simulink library "flight_dynamics_models"  (R2018b)
settings: Solver=VariableStepAuto  StartTime=0.0  StopTime=10.0  RelTol=1e-3
undefined symbols (not defined in the file or in its folder): aircraft, ic
libraries: vlm_wing_lib x12, flight_parameters_lib x4, axes_transformation_lib x4, fuselage_lib x4, wing_downwash_lib x4, se2a_actuators_lib x4, $bdroot x2, flexibleBody_lib x2, rigidBody_lib x2
(part 1 of 2)
settings Model: Creator=Ybeyer  LastModifiedBy=yannic
settings SFSimCC: SimUseLocalCustomCode=off
settings RTWCC: RTWUseLocalCustomCode=off
settings CodeAppCC: StateflowObjectComments=on

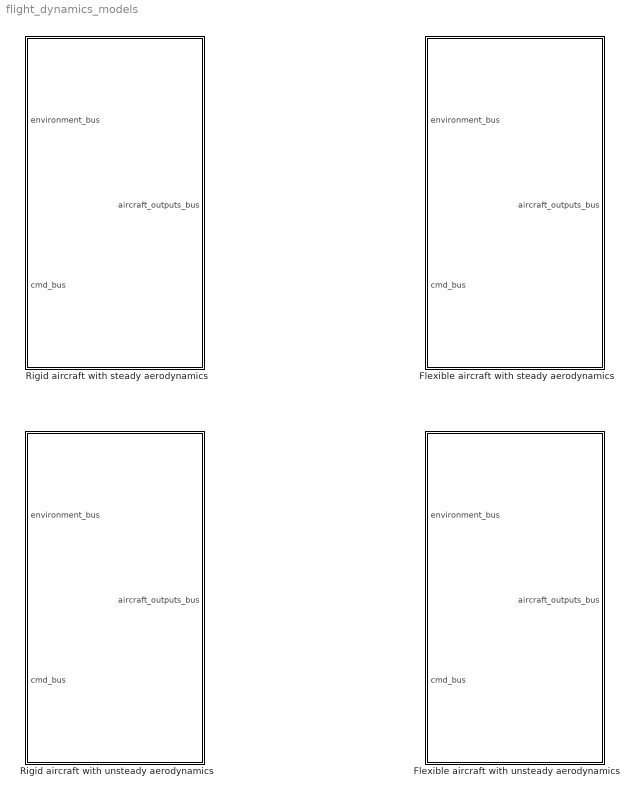
== system flight_dynamics_models ==
  Flexible aircraft with steady aerodynamics : Subsystem  mask{aircraft=aircraft, ic=ic}
      mask prompts: aircraft "Aircraft parameters struct, see aircraftSe2aCreate"; ic "Initial conditions struct"
      mask init:
      | aircraft_state = aircraftSe2aGetState(aircraft);
      | struct2bus(aircraft_state);
      mask DialogControl DescGroupVar Prompt: Rigid aircraft with steady aerodynamics
      mask DialogControl DescTextVar Prompt: Rigid body aerodynamics, steady aerodynamics based on nonlinear vortex step method, no unsteady aerodynamics.
      mask DialogControl Control2 Prompt: There are three wings: main wing, horizontal tailplane, vertical tailplane. There is no interaction between these wings. A simple fuselage model is used.
  Flexible aircraft with unsteady aerodynamics : Subsystem  mask{aircraft=aircraft, ic=ic}
      mask prompts: aircraft "aircraft parameters struct, see aircraftSe2aCreate"; ic "initial conditions struct"
      mask init:
      | aircraft_state = aircraftSe2aGetState(aircraft);
      | struct2bus(aircraft_state);
      mask DialogControl DescGroupVar Prompt: Rigid aircraft with steady aerodynamics
      mask DialogControl DescTextVar Prompt: Rigid body aerodynamics, steady aerodynamics based on nonlinear vortex step method, no unsteady aerodynamics.
      mask DialogControl Control2 Prompt: There are three wings: main wing, horizontal tailplane, vertical tailplane. There is no interaction between these wings. A simple fuselage model is used.
  Rigid aircraft with steady aerodynamics : Subsystem  mask{aircraft=aircraft, ic=ic}
      mask prompts: aircraft "Aircraft parameters struct, see aircraftSe2aCreate"; ic "Initial conditions struct"
      mask init:
      | aircraft_state = aircraftSe2aGetState(aircraft);
      | struct2bus(aircraft_state);
      mask DialogControl DescGroupVar Prompt: Rigid aircraft with steady aerodynamics
      mask DialogControl DescTextVar Prompt: Rigid body aerodynamics, steady aerodynamics based on nonlinear vortex step method, no unsteady aerodynamics.
      mask DialogControl Control2 Prompt: There are three wings: main wing, horizontal tailplane, vertical tailplane. There is no interaction between these wings. A simple fuselage model is used.
  Rigid aircraft with unsteady aerodynamics : Subsystem  mask{aircraft=aircraft, ic=ic}
      mask prompts: aircraft "Aircraft parameters struct, see aircraftSe2aCreate"; ic "Initial conditions struct"
      mask DialogControl DescGroupVar Prompt: Rigid aircraft with steady aerodynamics
      mask DialogControl DescTextVar Prompt: Rigid body aerodynamics, steady aerodynamics based on nonlinear vortex step method, no unsteady aerodynamics.
      mask DialogControl Control2 Prompt: There are three wings: main wing, horizontal tailplane, vertical tailplane. There is no interaction between these wings. A simple fuselage model is used.

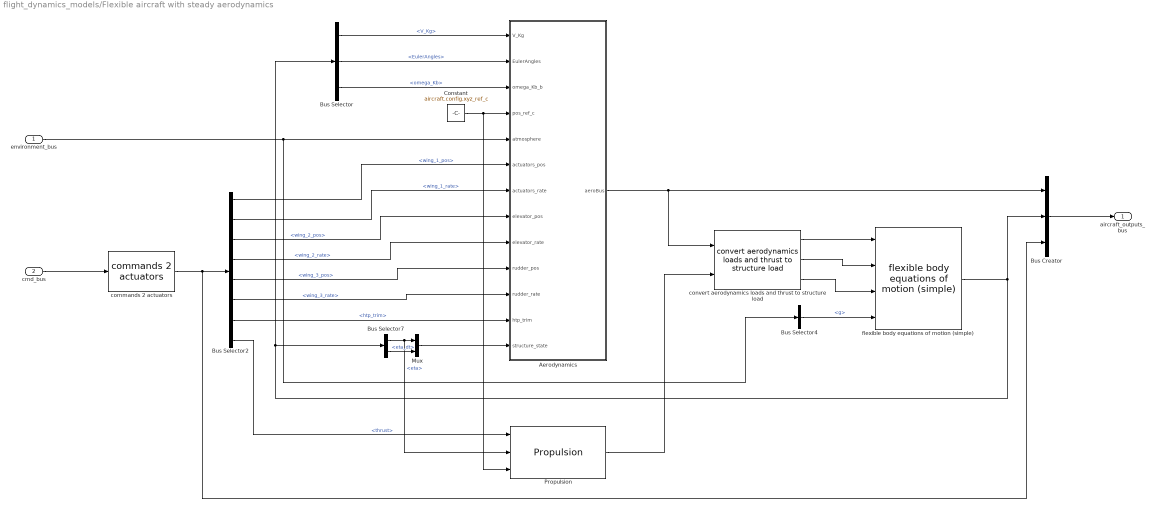
== system flight_dynamics_models/Flexible aircraft with steady aerodynamics ==
  environment_bus : Inport
  cmd_bus : Inport  Port=2
  Aerodynamics : Subsystem
  Bus Creator : BusCreator  Inputs=3
  Bus Selector : BusSelector  OutputSignals=rigidBodyBus.V_Kg,rigidBodyBus.EulerAngles,rigidBodyBus.omega_Kb
  Bus Selector2 : BusSelector  OutputSignals=wing_1_pos,wing_1_rate,wing_2_pos,wing_2_rate,wing_3_pos,wing_3_rate,htp_trim,thrust
  Bus Selector4 : BusSelector  OutputSignals=envir.g
  Bus Selector7 : BusSelector  OutputSignals=eta,eta_dt
  Constant : Constant  Value=aircraft.config.xyz_ref_c
  Mux : Mux  Inputs=2
  Propulsion : $bdroot/Flexible aircraft with unsteady aerodynamics/Propulsion  engines=aircraft.engines
  commands 2 actuators : se2a_actuators_lib/commands 2 actuators  aileron=aircraft.actuators.aileron  elevator=aircraft.actuators.elevator  rudder=aircraft.actuators.rudder  lads=aircraft.actuators.LAD  engines=aircraft.actuators.engines  htp_trim=aircraft.actuators.htp_trim
      settings: SourceProductName=SE2A library
  convert aerodynamics loads and thrust to structure load : $bdroot/Flexible aircraft with unsteady aerodynamics/convert aerodynamics loads  and thrust to structure load  SystemSampleTime=-1
  flexible body equations of motion (simple) : flexibleBody_lib/flexible body equations of motion (simple)  structure_red=aircraft.eom_flexible.structure_red  m=aircraft.eom_flexible.body.m  I_b=aircraft.eom_flexible.body.I  m_nodes=aircraft.eom_flexible.node_mass  cg_nodes=aircraft.eom_flexible.cg_nodes  structure_vel_0=zeros(size(aircraft.eom_flexible.structure_red.K,2)-6,1)  structure_pos_0=zeros(size(aircraft.eom_flexible.structure_red.K,2)-6,1)
      settings: SourceProductName=LADAC
  aircraft_outputs_bus : Outport
  wires:
  Bus Selector/1 -> Aerodynamics/1(V_Kg)  "<V_Kg>"
  Bus Selector/2 -> Aerodynamics/2(EulerAngles)  "<EulerAngles>"
  Bus Selector/3 -> Aerodynamics/3(omega_Kb_b)  "<omega_Kb>"
  Bus Creator/1 -> aircraft_outputs_bus/1
  Aerodynamics/1(aeroBus) -> convert aerodynamics loads and thrust to structure load/1, Bus Creator/1
  Bus Selector2/4 -> Aerodynamics/9(elevator_rate)  "<wing_2_rate>"
  Bus Selector2/5 -> Aerodynamics/10(rudder_pos)  "<wing_3_pos>"
  Bus Selector2/1 -> Aerodynamics/6(actuators_pos)  "<wing_1_pos>"
  Bus Selector2/2 -> Aerodynamics/7(actuators_rate)  "<wing_1_rate>"
  cmd_bus/1 -> commands 2 actuators/1
  Bus Selector2/7 -> Aerodynamics/12(htp_trim)  "<htp_trim>"
  Bus Selector2/3 -> Aerodynamics/8(elevator_pos)  "<wing_2_pos>"
  Bus Selector2/6 -> Aerodynamics/11(rudder_rate)  "<wing_3_rate>"
  Constant/1 -> Propulsion/3, Aerodynamics/4(pos_ref_c)
  Bus Selector4/1 -> flexible body equations of motion (simple)/4  "<g>"
  convert aerodynamics loads and thrust to structure load/1 -> flexible body equations of motion (simple)/1
  environment_bus/1 -> Bus Selector4/1, Aerodynamics/5(atmosphere)
  flexible body equations of motion (simple)/1 -> Bus Selector7/1, Bus Selector/1, Bus Creator/2
  Bus Selector7/2 -> Mux/2  "<eta_dt>"
  Mux/1 -> Aerodynamics/13(structure_state)
  Bus Selector7/1 -> Propulsion/2, Mux/1  "<eta>"
  Bus Selector2/8 -> Propulsion/1  "<thrust>"
  Propulsion/1 -> convert aerodynamics loads and thrust to structure load/2
  convert aerodynamics loads and thrust to structure load/3 -> flexible body equations of motion (simple)/3
  convert aerodynamics loads and thrust to structure load/2 -> flexible body equations of motion (simple)/2
  commands 2 actuators/1 -> Bus Creator/3, Bus Selector2/1

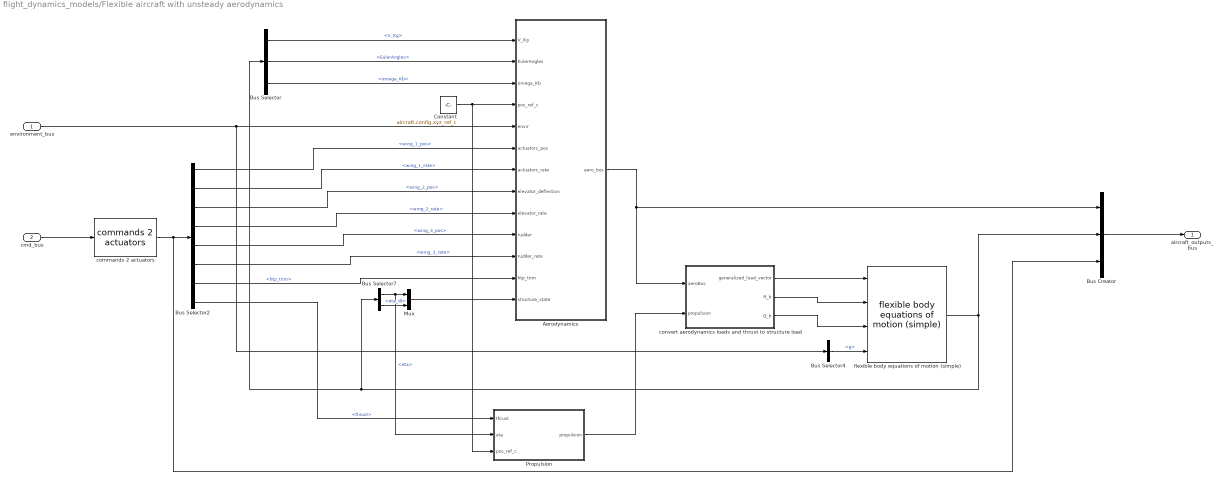
== system flight_dynamics_models/Flexible aircraft with unsteady aerodynamics ==
  environment_bus : Inport
  cmd_bus : Inport  Port=2
  Aerodynamics : Subsystem
  Bus Creator : BusCreator  Inputs=3
  Bus Selector : BusSelector  OutputSignals=rigidBodyBus.V_Kg,rigidBodyBus.EulerAngles,rigidBodyBus.omega_Kb
  Bus Selector2 : BusSelector  OutputSignals=wing_1_pos,wing_1_rate,wing_2_pos,wing_2_rate,wing_3_pos,wing_3_rate,htp_trim,thrust
  Bus Selector4 : BusSelector  OutputSignals=envir.g
  Bus Selector7 : BusSelector  OutputSignals=eta,eta_dt
  Constant : Constant  Value=aircraft.config.xyz_ref_c
  Mux : Mux  Inputs=2
  Propulsion : Subsystem  mask{engines=aircraft.engines}
      mask prompts: engines "engine parameters"
      mask DialogControl DescGroupVar Prompt: Propulsion
  commands 2 actuators : se2a_actuators_lib/commands 2 actuators  aileron=aircraft.actuators.aileron  elevator=aircraft.actuators.elevator  rudder=aircraft.actuators.rudder  lads=aircraft.actuators.LAD  engines=aircraft.actuators.engines  htp_trim=aircraft.actuators.htp_trim
      settings: SourceProductName=SE2A library
  convert aerodynamics loads and thrust to structure load : Subsystem
  flexible body equations of motion (simple) : flexibleBody_lib/flexible body equations of motion (simple)  structure_red=aircraft.eom_flexible.structure_red  m=aircraft.eom_flexible.body.m  I_b=aircraft.eom_flexible.body.I  m_nodes=aircraft.eom_flexible.node_mass  cg_nodes=aircraft.eom_flexible.cg_nodes  structure_vel_0=zeros(size(aircraft.eom_flexible.structure_red.K,2)-6,1)  structure_pos_0=zeros(size(aircraft.eom_flexible.structure_red.K,2)-6,1)
      settings: SourceProductName=LADAC
  aircraft_outputs_bus : Outport
  wires:
  Bus Selector4/1 -> flexible body equations of motion (simple)/4  "<g>"
  convert aerodynamics loads and thrust to structure load/1(generalized_load_vector) -> flexible body equations of motion (simple)/1
  flexible body equations of motion (simple)/1 -> Bus Creator/2, Bus Selector/1, Bus Selector7/1
  Aerodynamics/1(aero_bus) -> convert aerodynamics loads and thrust to structure load/1(aeroBus), Bus Creator/1
  Bus Selector2/7 -> Aerodynamics/12(htp_trim)  "<htp_trim>"
  Bus Selector2/5 -> Aerodynamics/10(rudder)  "<wing_3_pos>"
  Bus Selector2/3 -> Aerodynamics/8(elevator_deflection)  "<wing_2_pos>"
  Bus Selector2/1 -> Aerodynamics/6(actuators_pos)  "<wing_1_pos>"
  commands 2 actuators/1 -> Bus Creator/3, Bus Selector2/1
  Bus Selector/3 -> Aerodynamics/3(omega_Kb)  "<omega_Kb>"
  Bus Selector/2 -> Aerodynamics/2(EulerAngles)  "<EulerAngles>"
  Bus Selector/1 -> Aerodynamics/1(V_Kg)  "<V_Kg>"
  environment_bus/1 -> Aerodynamics/5(envir), Bus Selector4/1
  Bus Selector2/8 -> Propulsion/1(thrust)  "<thrust>"
  Bus Selector2/2 -> Aerodynamics/7(actuators_rate)  "<wing_1_rate>"
  Bus Selector2/4 -> Aerodynamics/9(elevator_rate)  "<wing_2_rate>"
  Bus Selector2/6 -> Aerodynamics/11(rudder_rate)  "<wing_3_rate>"
  Mux/1 -> Aerodynamics/13(structure_state)
  Bus Selector7/2 -> Mux/2  "<eta_dt>"
  Bus Selector7/1 -> Propulsion/2(eta), Mux/1  "<eta>"
  Constant/1 -> Propulsion/3(pos_ref_c), Aerodynamics/4(pos_ref_c)
  convert aerodynamics loads and thrust to structure load/2(R_b) -> flexible body equations of motion (simple)/2
  convert aerodynamics loads and thrust to structure load/3(Q_b) -> flexible body equations of motion (simple)/3
  Propulsion/1(propulsion) -> convert aerodynamics loads and thrust to structure load/2(propulsion)
  cmd_bus/1 -> commands 2 actuators/1
  Bus Creator/1 -> aircraft_outputs_bus/1

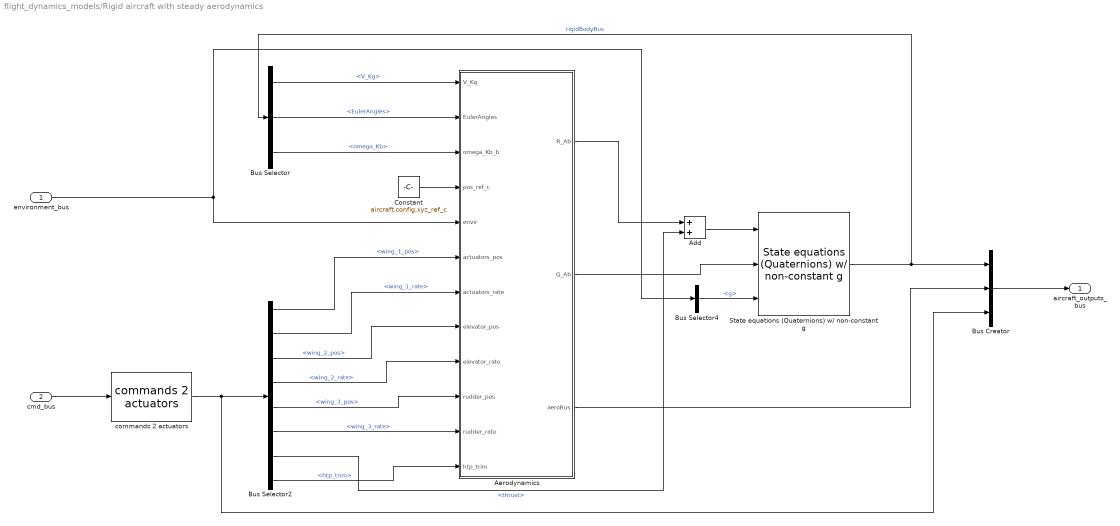
== system flight_dynamics_models/Rigid aircraft with steady aerodynamics ==
  environment_bus : Inport
  cmd_bus : Inport  Port=2
  Add : Sum
  Aerodynamics : Subsystem
  Bus Creator : BusCreator  Inputs=3
  Bus Selector : BusSelector  OutputSignals=V_Kg,EulerAngles,omega_Kb
  Bus Selector2 : BusSelector  OutputSignals=wing_1_pos,wing_1_rate,wing_2_pos,wing_2_rate,wing_3_pos,wing_3_rate,thrust,htp_trim
  Bus Selector4 : BusSelector  OutputSignals=envir.g
  Constant : Constant  Value=aircraft.config.xyz_ref_c
  State equations (Quaternions) w/ non-constant g : rigidBody_lib/State equations (Quaternions) w// non-constant g  mass=aircraft.eom_rigid.m  inertia=aircraft.eom_rigid.I  omega_Kb_0=ic.omega_Kb  q_bg_0=ic.q_bg  V_Kb_0=ic.V_Kb  s_g_0=ic.s_Kg
      settings: SourceProductName=LADAC
  commands 2 actuators : se2a_actuators_lib/commands 2 actuators  aileron=aircraft.actuators.aileron  elevator=aircraft.actuators.elevator  rudder=aircraft.actuators.rudder  lads=aircraft.actuators.LAD  engines=aircraft.actuators.engines  htp_trim=aircraft.actuators.htp_trim
      settings: SourceProductName=SE2A library
  aircraft_outputs_bus : Outport
  wires:
  Aerodynamics/2(Q_Ab) -> State equations (Quaternions) w/ non-constant g/2
  Aerodynamics/1(R_Ab) -> Add/1
  Add/1 -> State equations (Quaternions) w/ non-constant g/1
  environment_bus/1 -> Bus Selector4/1, Aerodynamics/5(envir)
  State equations (Quaternions) w/ non-constant g/1 -> Bus Selector/1, Bus Creator/1  "rigidBodyBus"
  Bus Selector/1 -> Aerodynamics/1(V_Kg)  "<V_Kg>"
  Bus Selector/2 -> Aerodynamics/2(EulerAngles)  "<EulerAngles>"
  Bus Selector/3 -> Aerodynamics/3(omega_Kb_b)  "<omega_Kb>"
  Bus Creator/1 -> aircraft_outputs_bus/1
  Aerodynamics/3(aeroBus) -> Bus Creator/2
  Bus Selector4/1 -> State equations (Quaternions) w/ non-constant g/3  "<g>"
  Bus Selector2/7 -> Add/2  "<thrust>"
  Bus Selector2/6 -> Aerodynamics/11(rudder_rate)  "<wing_3_rate>"
  Bus Selector2/8 -> Aerodynamics/12(htp_trim)  "<htp_trim>"
  Bus Selector2/3 -> Aerodynamics/8(elevator_pos)  "<wing_2_pos>"
  Bus Selector2/2 -> Aerodynamics/7(actuators_rate)  "<wing_1_rate>"
  cmd_bus/1 -> commands 2 actuators/1
  Bus Selector2/1 -> Aerodynamics/6(actuators_pos)  "<wing_1_pos>"
  Bus Selector2/5 -> Aerodynamics/10(rudder_pos)  "<wing_3_pos>"
  Bus Selector2/4 -> Aerodynamics/9(elevator_rate)  "<wing_2_rate>"
  Constant/1 -> Aerodynamics/4(pos_ref_c)
  commands 2 actuators/1 -> Bus Creator/3, Bus Selector2/1

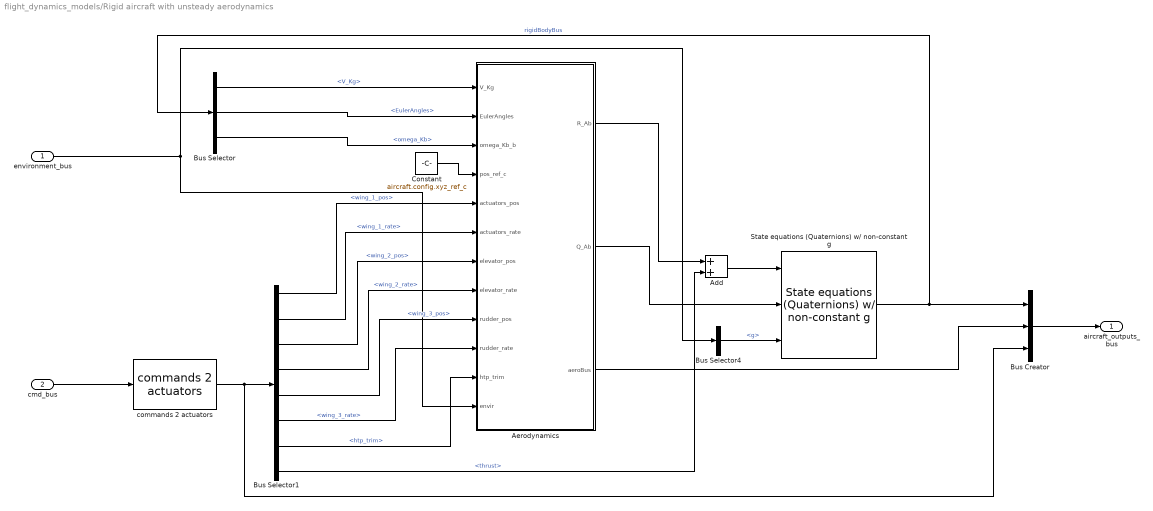
== system flight_dynamics_models/Rigid aircraft with unsteady aerodynamics ==
  environment_bus : Inport
  cmd_bus : Inport  Port=2
  Add : Sum
  Aerodynamics : Subsystem
  Bus Creator : BusCreator  Inputs=3
  Bus Selector : BusSelector  OutputSignals=V_Kg,EulerAngles,omega_Kb
  Bus Selector1 : BusSelector  OutputSignals=wing_1_pos,wing_1_rate,wing_2_pos,wing_2_rate,wing_3_pos,wing_3_rate,htp_trim,thrust
  Bus Selector4 : BusSelector  OutputSignals=g
  Constant : Constant  Value=aircraft.config.xyz_ref_c
  State equations (Quaternions) w/ non-constant g : rigidBody_lib/State equations (Quaternions) w// non-constant g  mass=aircraft.eom_rigid.m  inertia=aircraft.eom_rigid.I  omega_Kb_0=ic.omega_Kb  q_bg_0=ic.q_bg  V_Kb_0=ic.V_Kb  s_g_0=ic.s_Kg
      settings: SourceProductName=LADAC
  commands 2 actuators : se2a_actuators_lib/commands 2 actuators  aileron=aircraft.actuators.aileron  elevator=aircraft.actuators.elevator  rudder=aircraft.actuators.rudder  lads=aircraft.actuators.LAD  engines=aircraft.actuators.engines  htp_trim=aircraft.actuators.htp_trim
      settings: SourceProductName=SE2A library
  aircraft_outputs_bus : Outport
  wires:
  Aerodynamics/3(aeroBus) -> Bus Creator/2
  Bus Selector1/7 -> Aerodynamics/11(htp_trim)  "<htp_trim>"
  Bus Selector1/5 -> Aerodynamics/9(rudder_pos)  "<wing_3_pos>"
  Bus Selector1/3 -> Aerodynamics/7(elevator_pos)  "<wing_2_pos>"
  Bus Selector1/1 -> Aerodynamics/5(actuators_pos)  "<wing_1_pos>"
  cmd_bus/1 -> commands 2 actuators/1
  Bus Creator/1 -> aircraft_outputs_bus/1
  Bus Selector/3 -> Aerodynamics/3(omega_Kb_b)  "<omega_Kb>"
  Bus Selector/2 -> Aerodynamics/2(EulerAngles)  "<EulerAngles>"
  Bus Selector/1 -> Aerodynamics/1(V_Kg)  "<V_Kg>"
  State equations (Quaternions) w/ non-constant g/1 -> Bus Selector/1, Bus Creator/1  "rigidBodyBus"
  environment_bus/1 -> Aerodynamics/12(envir), Bus Selector4/1
  Bus Selector1/8 -> Add/2  "<thrust>"
  Add/1 -> State equations (Quaternions) w/ non-constant g/1
  Aerodynamics/1(R_Ab) -> Add/1
  Aerodynamics/2(Q_Ab) -> State equations (Quaternions) w/ non-constant g/2
  Bus Selector4/1 -> State equations (Quaternions) w/ non-constant g/3  "<g>"
  Bus Selector1/2 -> Aerodynamics/6(actuators_rate)  "<wing_1_rate>"
  Bus Selector1/4 -> Aerodynamics/8(elevator_rate)  "<wing_2_rate>"
  Bus Selector1/6 -> Aerodynamics/10(rudder_rate)  "<wing_3_rate>"
  Constant/1 -> Aerodynamics/4(pos_ref_c)
  commands 2 actuators/1 -> Bus Creator/3, Bus Selector1/1

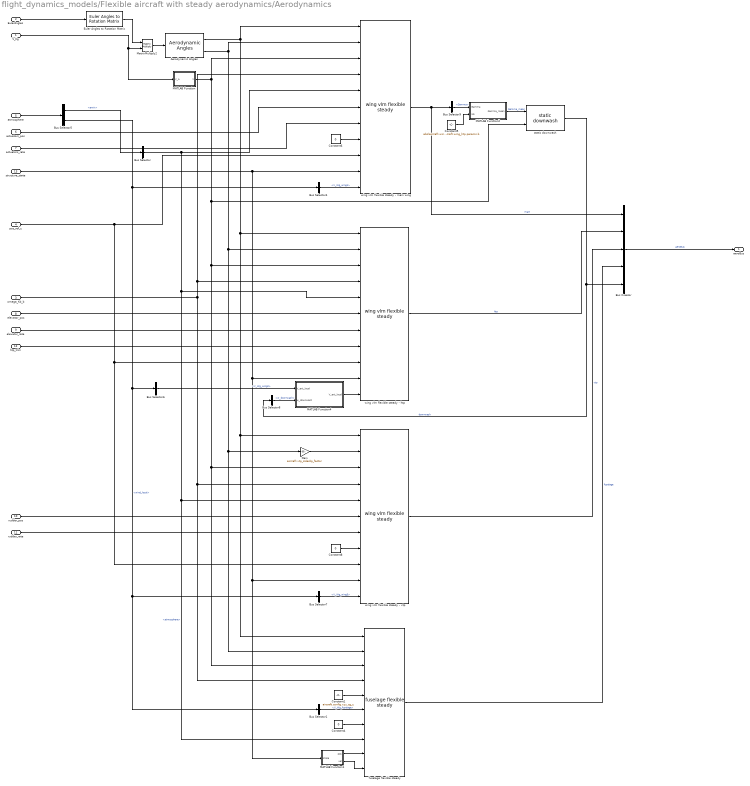
== system flight_dynamics_models/Flexible aircraft with steady aerodynamics/Aerodynamics ==
  V_Kg : Inport
  EulerAngles : Inport  Port=2
  omega_Kb_b : Inport  Port=3
  pos_ref_c : Inport  Port=4
  atmosphere : Inport  Port=5
  actuators_pos : Inport  Port=6
  actuators_rate : Inport  Port=7
  elevator_pos : Inport  Port=8
  elevator_rate : Inport  Port=9
  rudder_pos : Inport  Port=10
  rudder_rate : Inport  Port=11
  htp_trim : Inport  Port=12
  structure_state : Inport  Port=13
  Aerodynamic Angles : flight_parameters_lib/Aerodynamic Angles  SystemSampleTime=-1
      settings: SourceProductName=LADAC
  Bus Creator : BusCreator  Inputs=5
  Bus Selector : BusSelector  OutputSignals=atmosphere
  Bus Selector1 : BusSelector  OutputSignals=V_Wg_local.V_Wg_fuselage
  Bus Selector4 : BusSelector  OutputSignals=V_Wg_local.V_Wg_wing1
  Bus Selector5 : BusSelector  OutputSignals=envir,wind_local
  Bus Selector6 : BusSelector  OutputSignals=V_Wg_local.V_Wg_wing2
  Bus Selector7 : BusSelector  OutputSignals=V_Wg_local.V_Wg_wing3
  Bus Selector8 : BusSelector  OutputSignals=w_downwash
  Bus Selector9 : BusSelector  OutputSignals=aero.circulation.Gamma
  Constant1 : Constant  Value=aircraft.config.xyz_cg_c
  Constant4 : Constant  Value=0
  Constant5 : Constant  Value=abs(aircraft.wing_main.geometry.ctrl_pt.pos(2,:))<aircraft.wing_htp.params.b
  Constant6 : Constant  Value=0
  Constant8 : Constant  Value=0
  Euler Angles to Rotation Matrix : axes_transformation_lib/Euler Angles to Rotation Matrix  SystemSampleTime=-1
      settings: SourceProductName=LADAC
  Gain : Gain  Gain=aircraft.vtp_sideslip_factor
  MATLAB Function : MATLAB Function  TreatAsAtomicUnit=on
  MATLAB Function1 : MATLAB Function  TreatAsAtomicUnit=on
  MATLAB Function2 : MATLAB Function  TreatAsAtomicUnit=on
  MATLAB Function4 : MATLAB Function  TreatAsAtomicUnit=on
  MatrixMultiply2 : Product  Multiplication=Matrix(*)
  fuselage flexible steady : fuselage_lib/fuselage flexible steady  fuselage_struct=aircraft.fuselage  fuselage_state_bus=fuselage_1_state_bus
      settings: SourceProductName=LADAC
  static downwash : wing_downwash_lib/static downwash  downwash=aircraft.downwash
      settings: SourceProductName=SE2A library
  wing vlm flexible steady - htp : vlm_wing_lib/wing vlm flexible steady  wing_struct=aircraft.wing_htp  wing_state_bus=wing_2_state_bus  alpha_ind_init=0
      settings: SourceProductName=LADAC
  wing vlm flexible steady - main wing : vlm_wing_lib/wing vlm flexible steady  wing_struct=aircraft.wing_main  wing_state_bus=wing_1_state_bus  alpha_ind_init=0
      settings: SourceProductName=LADAC
  wing vlm flexible steady - vtp : vlm_wing_lib/wing vlm flexible steady  wing_struct=aircraft.wing_vtp  wing_state_bus=wing_3_state_bus  alpha_ind_init=0
      settings: SourceProductName=LADAC
  aeroBus : Outport
  wires:
  Euler Angles to Rotation Matrix/1 -> MatrixMultiply2/1
  EulerAngles/1 -> Euler Angles to Rotation Matrix/1
  V_Kg/1 -> MATLAB Function/1(V_A), MatrixMultiply2/2
  MatrixMultiply2/1 -> Aerodynamic Angles/1
  elevator_rate/1 -> wing vlm flexible steady - htp/7
  htp_trim/1 -> wing vlm flexible steady - htp/8
  wing vlm flexible steady - htp/1 -> Bus Creator/2  "htp"
  Bus Creator/1 -> aeroBus/1  "aeroBus"
  actuators_rate/1 -> wing vlm flexible steady - main wing/7
  Constant6/1 -> wing vlm flexible steady - main wing/8
  rudder_rate/1 -> wing vlm flexible steady - vtp/7
  Constant8/1 -> wing vlm flexible steady - vtp/8
  pos_ref_c/1 -> wing vlm flexible steady - vtp/9, wing vlm flexible steady - htp/9, wing vlm flexible steady - main wing/9
  wing vlm flexible steady - vtp/1 -> Bus Creator/3  "vtp"
  structure_state/1 -> MATLAB Function1/1(state), wing vlm flexible steady - vtp/10, wing vlm flexible steady - htp/10, wing vlm flexible steady - main wing/10
  Gain/1 -> wing vlm flexible steady - vtp/2
  actuators_pos/1 -> wing vlm flexible steady - main wing/6
  elevator_pos/1 -> wing vlm flexible steady - htp/6
  rudder_pos/1 -> wing vlm flexible steady - vtp/6
  atmosphere/1 -> Bus Selector5/1
  Bus Selector5/2 -> Bus Selector1/1, Bus Selector7/1, Bus Selector6/1, Bus Selector4/1  "<wind_local>"
  Bus Selector7/1 -> wing vlm flexible steady - vtp/11  "<V_Wg_wing3>"
  Bus Selector5/1 -> Bus Selector/1  "<envir>"
  Bus Selector4/1 -> wing vlm flexible steady - main wing/11  "<V_Wg_wing1>"
  Aerodynamic Angles/1 -> fuselage flexible steady/1, wing vlm flexible steady - vtp/1, wing vlm flexible steady - htp/1, wing vlm flexible steady - main wing/1
  Bus Selector1/1 -> fuselage flexible steady/6  "<V_Wg_fuselage>"
  MATLAB Function/1(V) -> wing vlm flexible steady - main wing/3, fuselage flexible steady/3, wing vlm flexible steady - vtp/3, wing vlm flexible steady - htp/3, static downwash/2
  Constant4/1 -> fuselage flexible steady/7
  fuselage flexible steady/1 -> Bus Creator/4  "fuselage"
  Constant1/1 -> fuselage flexible steady/5
  Bus Selector/1 -> wing vlm flexible steady - main wing/5, fuselage flexible steady/8, wing vlm flexible steady - vtp/5, wing vlm flexible steady - htp/5  "<atmosphere>"
  omega_Kb_b/1 -> wing vlm flexible steady - htp/4, wing vlm flexible steady - main wing/4, fuselage flexible steady/4, wing vlm flexible steady - vtp/4
  Aerodynamic Angles/2 -> fuselage flexible steady/2, Gain/1, wing vlm flexible steady - htp/2, wing vlm flexible steady - main wing/2
  MATLAB Function1/1(pos) -> fuselage flexible steady/9
  MATLAB Function1/2(vel) -> fuselage flexible steady/10
  Constant5/1 -> MATLAB Function2/2(idx)
  Bus Selector9/1 -> MATLAB Function2/1(Gamma)  "<Gamma>"
  MATLAB Function2/1(Gamma_mean) -> static downwash/1  "Gamma_mean"
  wing vlm flexible steady - main wing/1 -> Bus Selector9/1, Bus Creator/1  "main"
  static downwash/1 -> Bus Selector8/1, Bus Creator/5  "downwash"
  Bus Selector6/1 -> MATLAB Function4/1("V_ext_local ")  "<V_Wg_wing2>"
  Bus Selector8/1 -> MATLAB Function4/2(w_downwash)  "<w_downwash>"
  MATLAB Function4/1(V_ext_local) -> wing vlm flexible steady - htp/11

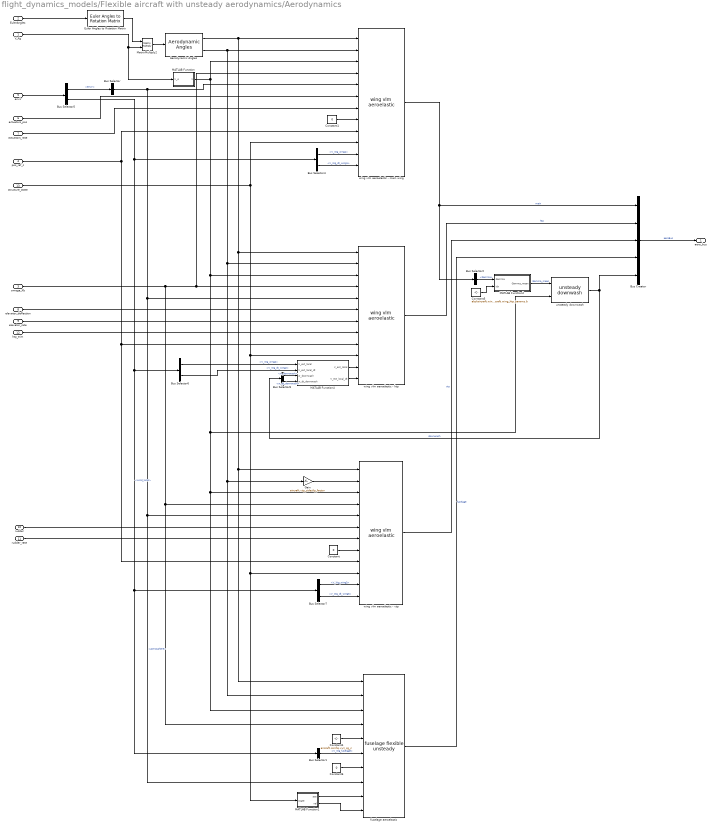
== system flight_dynamics_models/Flexible aircraft with unsteady aerodynamics/Aerodynamics ==
  V_Kg : Inport
  EulerAngles : Inport  Port=2
  omega_Kb : Inport  Port=3
  pos_ref_c : Inport  Port=4
  envir : Inport  Port=5
  actuators_pos : Inport  Port=6
  actuators_rate : Inport  Port=7
  elevator_deflection : Inport  Port=8
  elevator_rate : Inport  Port=9
  rudder : Inport  Port=10
  rudder_rate : Inport  Port=11
  htp_trim : Inport  Port=12
  structure_state : Inport  Port=13
  Aerodynamic Angles : flight_parameters_lib/Aerodynamic Angles  SystemSampleTime=-1
      settings: SourceProductName=LADAC
  Bus Creator : BusCreator  Inputs=5
  Bus Selector : BusSelector  OutputSignals=atmosphere
  Bus Selector1 : BusSelector  OutputSignals=V_Wg_local.V_Wg_fuselage
  Bus Selector2 : BusSelector  OutputSignals=aero.circulation.Gamma
  Bus Selector4 : BusSelector  OutputSignals=V_Wg_local.V_Wg_wing1,V_Wg_dt_local.V_Wg_dt_wing1
  Bus Selector5 : BusSelector  OutputSignals=envir,wind_local
  Bus Selector6 : BusSelector  OutputSignals=V_Wg_local.V_Wg_wing2,V_Wg_dt_local.V_Wg_dt_wing2
  Bus Selector7 : BusSelector  OutputSignals=V_Wg_local.V_Wg_wing3,V_Wg_dt_local.V_Wg_dt_wing3
  Bus Selector8 : BusSelector  OutputSignals=w_downwash,w_dt_downwash
  Constant : Constant  Value=0
  Constant1 : Constant  Value=0
  Constant4 : Constant  Value=aircraft.config.xyz_cg_c
  Constant5 : Constant  Value=abs(aircraft.wing_main.geometry.ctrl_pt.pos(2,:))<aircraft.wing_htp.params.b
  Constant6 : Constant  Value=0
  Euler Angles to Rotation Matrix : axes_transformation_lib/Euler Angles to Rotation Matrix  SystemSampleTime=-1
      settings: SourceProductName=LADAC
  Gain : Gain  Gain=aircraft.vtp_sideslip_factor
  MATLAB Function : MATLAB Function  TreatAsAtomicUnit=on
  MATLAB Function1 : MATLAB Function  TreatAsAtomicUnit=on
  MATLAB Function2 : MATLAB Function  TreatAsAtomicUnit=on
  MATLAB Function4 : MATLAB Function  TreatAsAtomicUnit=on
  MatrixMultiply2 : Product  Multiplication=Matrix(*)
  fuselage aeroelastic : fuselage_lib/fuselage flexible unsteady  fuselage_struct=aircraft.fuselage  fuselage_state_bus=fuselage_1_state_bus
      settings: SourceProductName=LADAC
  unsteady downwash : wing_downwash_lib/unsteady downwash  downwash=aircraft.downwash
      settings: SourceProductName=LADAC
  wing vlm aeroelastic - htp : vlm_wing_lib/wing vlm aeroelastic  wing_struct=aircraft.wing_htp  wing_state_bus=wing_2_state_bus  unst_aero_state_init=0  dyn_stall_state_init=0  unst_flap_state_init=0  unst_act2_state_init=0  tau_v_init=0  alpha_ind_init=0
      settings: SourceProductName=LADAC
  wing vlm aeroelastic - main wing : vlm_wing_lib/wing vlm aeroelastic  wing_struct=aircraft.wing_main  wing_state_bus=wing_1_state_bus  unst_aero_state_init=0  dyn_stall_state_init=0  unst_flap_state_init=0  unst_act2_state_init=0  tau_v_init=0  alpha_ind_init=0
      settings: SourceProductName=LADAC
  wing vlm aeroelastic - vtp : vlm_wing_lib/wing vlm aeroelastic  wing_struct=aircraft.wing_vtp  wing_state_bus=wing_3_state_bus  unst_aero_state_init=0  dyn_stall_state_init=0  unst_flap_state_init=0  unst_act2_state_init=0  tau_v_init=0  alpha_ind_init=0
      settings: SourceProductName=LADAC
  aero_bus : Outport
  wires:
  Bus Selector7/2 -> wing vlm aeroelastic - vtp/12  "<V_Wg_dt_wing3>"
  Bus Selector7/1 -> wing vlm aeroelastic - vtp/11  "<V_Wg_wing3>"
  Bus Selector6/2 -> MATLAB Function4/2("V_ext_local_dt ")  "<V_Wg_dt_wing2>"
  Bus Selector6/1 -> MATLAB Function4/1("V_ext_local ")  "<V_Wg_wing2>"
  Bus Selector4/1 -> wing vlm aeroelastic - main wing/11  "<V_Wg_wing1>"
  Bus Selector4/2 -> wing vlm aeroelastic - main wing/12  "<V_Wg_dt_wing1>"
  Bus Selector5/2 -> Bus Selector1/1, Bus Selector7/1, Bus Selector6/1, Bus Selector4/1  "<wind_local>"
  envir/1 -> Bus Selector5/1
  wing vlm aeroelastic - vtp/1 -> Bus Creator/3  "vtp"
  wing vlm aeroelastic - htp/1 -> Bus Creator/2  "htp"
  rudder/1 -> wing vlm aeroelastic - vtp/6
  wing vlm aeroelastic - main wing/1 -> Bus Selector2/1, Bus Creator/1  "main"
  actuators_pos/1 -> wing vlm aeroelastic - main wing/6
  Bus Creator/1 -> aero_bus/1  "aeroBus"
  htp_trim/1 -> wing vlm aeroelastic - htp/8
  elevator_deflection/1 -> wing vlm aeroelastic - htp/6
  MatrixMultiply2/1 -> Aerodynamic Angles/1
  V_Kg/1 -> MatrixMultiply2/2, MATLAB Function/1(V_A)
  Bus Selector5/1 -> Bus Selector/1  "<envir>"
  EulerAngles/1 -> Euler Angles to Rotation Matrix/1
  Euler Angles to Rotation Matrix/1 -> MatrixMultiply2/1
  elevator_rate/1 -> wing vlm aeroelastic - htp/7
  actuators_rate/1 -> wing vlm aeroelastic - main wing/7
  rudder_rate/1 -> wing vlm aeroelastic - vtp/7
  Constant/1 -> wing vlm aeroelastic - vtp/8
  Constant1/1 -> wing vlm aeroelastic - main wing/8
  pos_ref_c/1 -> wing vlm aeroelastic - main wing/9, wing vlm aeroelastic - vtp/9, wing vlm aeroelastic - htp/9
  Gain/1 -> wing vlm aeroelastic - vtp/2
  Constant6/1 -> fuselage aeroelastic/7
  Constant4/1 -> fuselage aeroelastic/5
  fuselage aeroelastic/1 -> Bus Creator/4  "fuselage"
  Bus Selector1/1 -> fuselage aeroelastic/6  "<V_Wg_fuselage>"
  Bus Selector/1 -> fuselage aeroelastic/8, wing vlm aeroelastic - vtp/5, wing vlm aeroelastic - htp/5, wing vlm aeroelastic - main wing/5  "<atmosphere>"
  structure_state/1 -> wing vlm aeroelastic - main wing/10, MATLAB Function1/1(state), wing vlm aeroelastic - vtp/10, wing vlm aeroelastic - htp/10
  MATLAB Function1/1(pos) -> fuselage aeroelastic/9
  MATLAB Function1/2(vel) -> fuselage aeroelastic/10
  Aerodynamic Angles/1 -> fuselage aeroelastic/1, wing vlm aeroelastic - vtp/1, wing vlm aeroelastic - htp/1, wing vlm aeroelastic - main wing/1
  Aerodynamic Angles/2 -> fuselage aeroelastic/2, Gain/1, wing vlm aeroelastic - htp/2, wing vlm aeroelastic - main wing/2
  omega_Kb/1 -> fuselage aeroelastic/4, wing vlm aeroelastic - vtp/4, wing vlm aeroelastic - htp/4, wing vlm aeroelastic - main wing/4
  Bus Selector2/1 -> MATLAB Function2/1(Gamma)  "<Gamma>"
  Constant5/1 -> MATLAB Function2/2(idx)
  MATLAB Function/1(V) -> unsteady downwash/2, fuselage aeroelastic/3, wing vlm aeroelastic - vtp/3, wing vlm aeroelastic - htp/3, wing vlm aeroelastic - main wing/3
  MATLAB Function4/1(V_ext_local) -> wing vlm aeroelastic - htp/11
  MATLAB Function4/2(V_ext_local_dt) -> wing vlm aeroelastic - htp/12
  Bus Selector8/1 -> MATLAB Function4/3(w_downwash)  "<w_downwash>"
  Bus Selector8/2 -> MATLAB Function4/4(w_dt_downwash)  "<w_dt_downwash>"
  unsteady downwash/1 -> Bus Selector8/1, Bus Creator/5  "downwash"
  MATLAB Function2/1(Gamma_mean) -> unsteady downwash/1  "Gamma_mean"

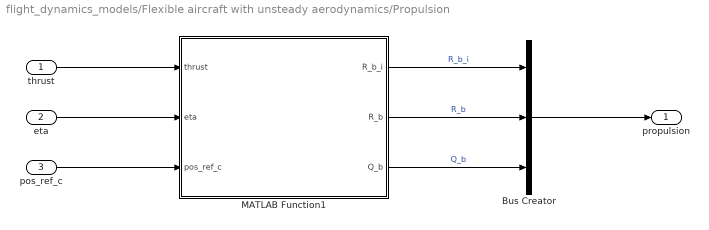
== system flight_dynamics_models/Flexible aircraft with unsteady aerodynamics/Propulsion ==
  thrust : Inport
  eta : Inport  Port=2
  pos_ref_c : Inport  Port=3
  Bus Creator : BusCreator  Inputs=3
  MATLAB Function1 : MATLAB Function  TreatAsAtomicUnit=on
  propulsion : Outport
  wires:
  Bus Creator/1 -> propulsion/1
  thrust/1 -> MATLAB Function1/1(thrust)
  eta/1 -> MATLAB Function1/2(eta)
  pos_ref_c/1 -> MATLAB Function1/3(pos_ref_c)
  MATLAB Function1/1(R_b_i) -> Bus Creator/1  "R_b_i"
  MATLAB Function1/2(R_b) -> Bus Creator/2  "R_b"
  MATLAB Function1/3(Q_b) -> Bus Creator/3  "Q_b"

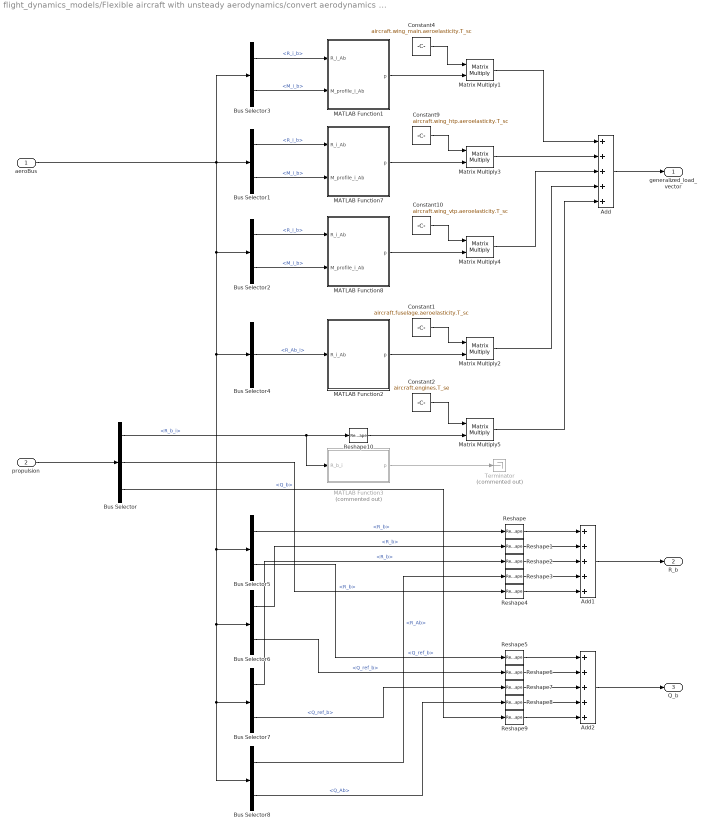
== system flight_dynamics_models/Flexible aircraft with unsteady aerodynamics/convert aerodynamics loads and thrust to structure load ==
  aeroBus : Inport
  propulsion : Inport  Port=2
  Add : Sum  Inputs=+++++
  Add1 : Sum  Inputs=+++++
  Add2 : Sum  Inputs=+++++
  Bus Selector : BusSelector  OutputSignals=R_b_i,R_b,Q_b
  Bus Selector1 : BusSelector  OutputSignals=htp.aero.force_loc.R_i_b,htp.aero.force_loc.M_i_b
  Bus Selector2 : BusSelector  OutputSignals=vtp.aero.force_loc.R_i_b,vtp.aero.force_loc.M_i_b
  Bus Selector3 : BusSelector  OutputSignals=main.aero.force_loc.R_i_b,main.aero.force_loc.M_i_b
  Bus Selector4 : BusSelector  OutputSignals=fuselage.aero.R_Ab_i
  Bus Selector5 : BusSelector  OutputSignals=main.aero.force_glob.R_b,main.aero.force_glob.Q_ref_b
  Bus Selector6 : BusSelector  OutputSignals=htp.aero.force_glob.R_b,htp.aero.force_glob.Q_ref_b
  Bus Selector7 : BusSelector  OutputSignals=vtp.aero.force_glob.R_b,vtp.aero.force_glob.Q_ref_b
  Bus Selector8 : BusSelector  OutputSignals=fuselage.aero.R_Ab,fuselage.aero.Q_Ab
  Constant1 : Constant  Value=aircraft.fuselage.aeroelasticity.T_sc
  Constant10 : Constant  Value=aircraft.wing_vtp.aeroelasticity.T_sc
  Constant2 : Constant  Value=aircraft.engines.T_se
  Constant4 : Constant  Value=aircraft.wing_main.aeroelasticity.T_sc
  Constant9 : Constant  Value=aircraft.wing_htp.aeroelasticity.T_sc
  MATLAB Function1 : MATLAB Function  TreatAsAtomicUnit=on
  MATLAB Function2 : MATLAB Function  TreatAsAtomicUnit=on
  MATLAB Function3 : MATLAB Function  Commented=on  TreatAsAtomicUnit=on
  MATLAB Function7 : MATLAB Function  TreatAsAtomicUnit=on
  MATLAB Function8 : MATLAB Function  TreatAsAtomicUnit=on
  Matrix Multiply{1..5} (5 alike) : Product  Multiplication=Matrix(*)
  Reshape{,1..9} (10 alike) : Reshape  OutputDimensionality=Column vector (2-D)
  Reshape10 : Reshape
  Terminator : Terminator  Commented=on
  generalized_load_vector : Outport
  R_b : Outport  Port=2
  Q_b : Outport  Port=3
  wires:
  Add/1 -> generalized_load_vector/1
  Matrix Multiply3/1 -> Add/2
  Matrix Multiply1/1 -> Add/1
  Constant4/1 -> Matrix Multiply1/1
  Bus Selector2/1 -> MATLAB Function8/1(R_i_Ab)  "<R_i_b>"
  MATLAB Function7/1(p) -> Matrix Multiply3/2
  Constant9/1 -> Matrix Multiply3/1
  Constant10/1 -> Matrix Multiply4/1
  Matrix Multiply4/1 -> Add/3
  Bus Selector1/2 -> MATLAB Function7/2(M_profile_i_Ab)  "<M_i_b>"
  Bus Selector1/1 -> MATLAB Function7/1(R_i_Ab)  "<R_i_b>"
  MATLAB Function1/1(p) -> Matrix Multiply1/2
  Bus Selector2/2 -> MATLAB Function8/2(M_profile_i_Ab)  "<M_i_b>"
  Bus Selector3/2 -> MATLAB Function1/2(M_profile_i_Ab)  "<M_i_b>"
  MATLAB Function8/1(p) -> Matrix Multiply4/2
  aeroBus/1 -> Bus Selector1/1, Bus Selector8/1, Bus Selector7/1, Bus Selector6/1, Bus Selector5/1, Bus Selector4/1, Bus Selector2/1, Bus Selector3/1
  Bus Selector3/1 -> MATLAB Function1/1(R_i_Ab)  "<R_i_b>"
  Bus Selector4/1 -> MATLAB Function2/1(R_i_Ab)  "<R_Ab_i>"
  MATLAB Function2/1(p) -> Matrix Multiply2/2
  Constant1/1 -> Matrix Multiply2/1
  Matrix Multiply2/1 -> Add/4
  propulsion/1 -> Bus Selector/1
  Constant2/1 -> Matrix Multiply5/1
  Matrix Multiply5/1 -> Add/5
  Bus Selector5/1 -> Reshape/1  "<R_b>"
  Bus Selector6/1 -> Reshape1/1  "<R_b>"
  Bus Selector7/1 -> Reshape2/1  "<R_b>"
  Bus Selector8/1 -> Reshape3/1  "<R_Ab>"
  Bus Selector5/2 -> Reshape5/1  "<Q_ref_b>"
  Bus Selector6/2 -> Reshape6/1  "<Q_ref_b>"
  Bus Selector7/2 -> Reshape7/1  "<Q_ref_b>"
  Bus Selector8/2 -> Reshape8/1  "<Q_Ab>"
  Add1/1 -> R_b/1
  Add2/1 -> Q_b/1
  Bus Selector/1 -> Reshape10/1, MATLAB Function3/1(R_b_i)  "<R_b_i>"
  Bus Selector/2 -> Reshape4/1  "<R_b>"
  Bus Selector/3 -> Reshape9/1  "<Q_b>"
  Reshape/1 -> Add1/1
  Reshape1/1 -> Add1/2
  Reshape2/1 -> Add1/3
  Reshape3/1 -> Add1/4
  Reshape4/1 -> Add1/5
  Reshape5/1 -> Add2/1
  Reshape6/1 -> Add2/2
  Reshape7/1 -> Add2/3
  Reshape8/1 -> Add2/4
  Reshape9/1 -> Add2/5
  MATLAB Function3/1(p) -> Terminator/1
  Reshape10/1 -> Matrix Multiply5/2

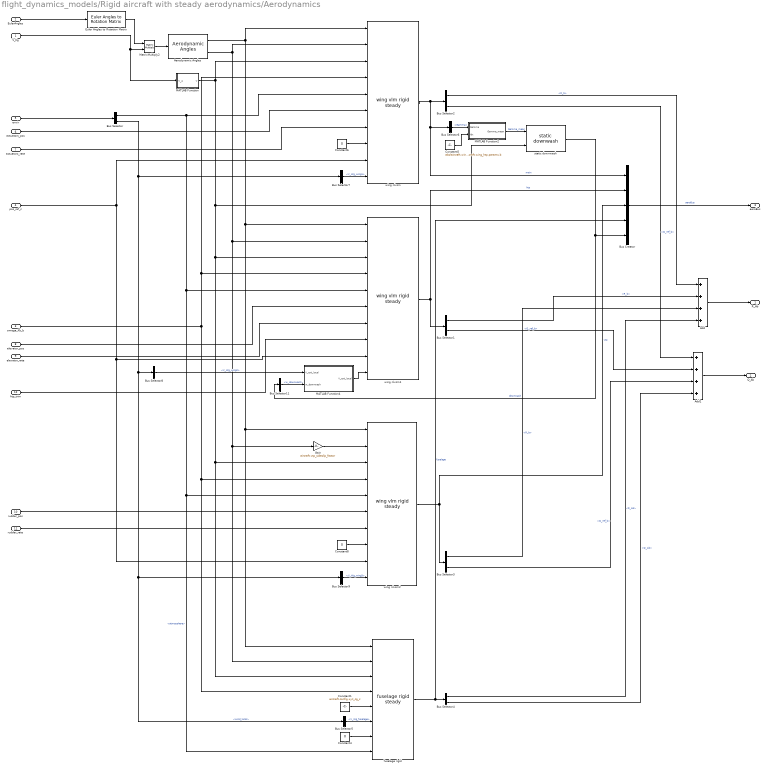
== system flight_dynamics_models/Rigid aircraft with steady aerodynamics/Aerodynamics ==
  V_Kg : Inport
  EulerAngles : Inport  Port=2
  omega_Kb_b : Inport  Port=3
  pos_ref_c : Inport  Port=4
  envir : Inport  Port=5
  actuators_pos : Inport  Port=6
  actuators_rate : Inport  Port=7
  elevator_pos : Inport  Port=8
  elevator_rate : Inport  Port=9
  rudder_pos : Inport  Port=10
  rudder_rate : Inport  Port=11
  htp_trim : Inport  Port=12
  Add : Sum  Inputs=++++
  Add1 : Sum  Inputs=++++
  Aerodynamic Angles : flight_parameters_lib/Aerodynamic Angles  SystemSampleTime=-1
      settings: SourceProductName=LADAC
  Bus Creator : BusCreator  Inputs=5
  Bus Selector : BusSelector  OutputSignals=envir.atmosphere,wind_local
  Bus Selector1 : BusSelector  OutputSignals=aero.force_glob.R_b,aero.force_glob.Q_ref_b
  Bus Selector11 : BusSelector  OutputSignals=w_downwash
  Bus Selector2 : BusSelector  OutputSignals=aero.force_glob.R_b,aero.force_glob.Q_ref_b
  Bus Selector3 : BusSelector  OutputSignals=aero.force_glob.R_b,aero.force_glob.Q_ref_b
  Bus Selector4 : BusSelector  OutputSignals=aero.R_Ab,aero.Q_Ab
  Bus Selector5 : BusSelector  OutputSignals=V_Wg_local.V_Wg_fuselage
  Bus Selector6 : BusSelector  OutputSignals=aero.circulation.Gamma
  Bus Selector7 : BusSelector  OutputSignals=V_Wg_local.V_Wg_wing1
  Bus Selector8 : BusSelector  OutputSignals=V_Wg_local.V_Wg_wing2
  Bus Selector9 : BusSelector  OutputSignals=V_Wg_local.V_Wg_wing3
  Constant1 : Constant  Value=aircraft.config.xyz_cg_c
  Constant4 : Constant  Value=0
  Constant5 : Constant  Value=abs(aircraft.wing_main.geometry.ctrl_pt.pos(2,:))<aircraft.wing_htp.params.b
  Constant6 : Constant  Value=0
  Constant8 : Constant  Value=0
  Euler Angles to Rotation Matrix : axes_transformation_lib/Euler Angles to Rotation Matrix  SystemSampleTime=-1
      settings: SourceProductName=LADAC
  Gain : Gain  Gain=aircraft.vtp_sideslip_factor
  MATLAB Function : MATLAB Function  TreatAsAtomicUnit=on
  MATLAB Function2 : MATLAB Function  TreatAsAtomicUnit=on
  MATLAB Function4 : MATLAB Function  TreatAsAtomicUnit=on
  MatrixMultiply2 : Product  Multiplication=Matrix(*)
  fuselage rigid : fuselage_lib/fuselage rigid steady  fuselage_struct=aircraft.fuselage  fuselage_state_bus=fuselage_1_state_bus
      settings: SourceProductName=LADAC
  static downwash : wing_downwash_lib/static downwash  downwash=aircraft.downwash
      settings: SourceProductName=LADAC
  wing nlvsm : vlm_wing_lib/wing vlm rigid steady  wing_struct=aircraft.wing_main  wing_state_bus=wing_1_state_bus  alpha_ind_init=0
      settings: SourceProductName=LADAC
  wing nlvsm1 : vlm_wing_lib/wing vlm rigid steady  wing_struct=aircraft.wing_htp  wing_state_bus=wing_2_state_bus  alpha_ind_init=0
      settings: SourceProductName=LADAC
  wing nlvsm2 : vlm_wing_lib/wing vlm rigid steady  wing_struct=aircraft.wing_vtp  wing_state_bus=wing_3_state_bus  alpha_ind_init=0
      settings: SourceProductName=LADAC
  R_Ab : Outport
  Q_Ab : Outport  Port=2
  aeroBus : Outport  Port=3
  wires:
  Bus Selector/2 -> Bus Selector5/1, Bus Selector9/1, Bus Selector8/1, Bus Selector7/1  "<wind_local>"
  envir/1 -> Bus Selector/1
  Euler Angles to Rotation Matrix/1 -> MatrixMultiply2/1
  EulerAngles/1 -> Euler Angles to Rotation Matrix/1
  Aerodynamic Angles/1 -> fuselage rigid/1, wing nlvsm2/1, wing nlvsm1/1, wing nlvsm/1
  Bus Selector/1 -> wing nlvsm/5, fuselage rigid/8, wing nlvsm2/5, wing nlvsm1/5  "<atmosphere>"
  Add/1 -> R_Ab/1
  Add1/1 -> Q_Ab/1
  V_Kg/1 -> MATLAB Function/1(V_A), MatrixMultiply2/2
  MatrixMultiply2/1 -> Aerodynamic Angles/1
  Bus Selector1/2 -> Add1/2  "<Q_ref_b>"
  Bus Selector1/1 -> Add/2  "<R_b>"
  elevator_pos/1 -> wing nlvsm1/6
  htp_trim/1 -> wing nlvsm1/8
  Bus Creator/1 -> aeroBus/1  "aeroBus"
  actuators_pos/1 -> wing nlvsm/6
  Constant6/1 -> wing nlvsm/8
  Bus Selector2/1 -> Add/1  "<R_b>"
  Bus Selector2/2 -> Add1/1  "<Q_ref_b>"
  rudder_pos/1 -> wing nlvsm2/6
  Constant8/1 -> wing nlvsm2/8
  pos_ref_c/1 -> wing nlvsm/9, wing nlvsm2/9, wing nlvsm1/9
  wing nlvsm2/1 -> Bus Selector3/1, Bus Creator/3  "vtp"
  Bus Selector3/1 -> Add/3  "<R_b>"
  Bus Selector3/2 -> Add1/3  "<Q_ref_b>"
  omega_Kb_b/1 -> wing nlvsm/4, wing nlvsm1/4, fuselage rigid/4, wing nlvsm2/4
  Bus Selector7/1 -> wing nlvsm/10  "<V_Wg_wing1>"
  Bus Selector9/1 -> wing nlvsm2/10  "<V_Wg_wing3>"
  wing nlvsm1/1 -> Bus Selector1/1, Bus Creator/2  "htp"
  rudder_rate/1 -> wing nlvsm2/7
  actuators_rate/1 -> wing nlvsm/7
  elevator_rate/1 -> wing nlvsm1/7
  Bus Selector5/1 -> fuselage rigid/6  "<V_Wg_fuselage>"
  Constant4/1 -> fuselage rigid/7
  fuselage rigid/1 -> Bus Creator/4, Bus Selector4/1  "fuselage"
  Bus Selector4/1 -> Add/4  "<R_Ab>"
  Constant1/1 -> fuselage rigid/5
  Bus Selector4/2 -> Add1/4  "<Q_Ab>"
  Aerodynamic Angles/2 -> fuselage rigid/2, Gain/1, wing nlvsm1/2, wing nlvsm/2
  Gain/1 -> wing nlvsm2/2
  MATLAB Function/1(V) -> wing nlvsm/3, fuselage rigid/3, wing nlvsm2/3, wing nlvsm1/3, static downwash/2
  MATLAB Function4/1(V_ext_local) -> wing nlvsm1/10
  MATLAB Function2/1(Gamma_mean) -> static downwash/1  "Gamma_mean"
  Bus Selector8/1 -> MATLAB Function4/1("V_ext_local ")  "<V_Wg_wing2>"
  static downwash/1 -> Bus Selector11/1, Bus Creator/5  "downwash"
  wing nlvsm/1 -> Bus Selector6/1, Bus Creator/1, Bus Selector2/1  "main"
  Constant5/1 -> MATLAB Function2/2(idx)
  Bus Selector6/1 -> MATLAB Function2/1(Gamma)  "<Gamma>"
  Bus Selector11/1 -> MATLAB Function4/2(w_downwash)  "<w_downwash>"

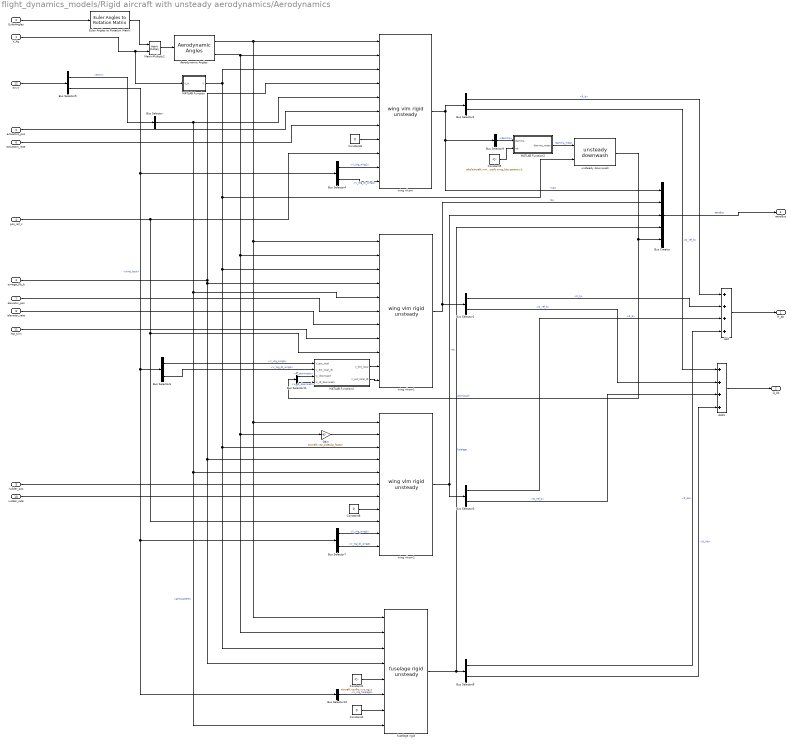
== system flight_dynamics_models/Rigid aircraft with unsteady aerodynamics/Aerodynamics ==
  V_Kg : Inport
  EulerAngles : Inport  Port=2
  omega_Kb_b : Inport  Port=3
  pos_ref_c : Inport  Port=4
  actuators_pos : Inport  Port=5
  actuators_rate : Inport  Port=6
  elevator_pos : Inport  Port=7
  elevator_rate : Inport  Port=8
  rudder_pos : Inport  Port=9
  rudder_rate : Inport  Port=10
  htp_trim : Inport  Port=11
  envir : Inport  Port=12
  Add : Sum  Inputs=++++
  Add1 : Sum  Inputs=++++
  Aerodynamic Angles : flight_parameters_lib/Aerodynamic Angles  SystemSampleTime=-1
      settings: SourceProductName=LADAC
  Bus Creator : BusCreator  Inputs=5
  Bus Selector : BusSelector  OutputSignals=atmosphere
  Bus Selector1 : BusSelector  OutputSignals=aero.force_glob.R_b,aero.force_glob.Q_ref_b
  Bus Selector10 : BusSelector  OutputSignals=V_Wg_local.V_Wg_fuselage
  Bus Selector11 : BusSelector  OutputSignals=w_downwash,w_dt_downwash
  Bus Selector2 : BusSelector  OutputSignals=aero.force_glob.R_b,aero.force_glob.Q_ref_b
  Bus Selector3 : BusSelector  OutputSignals=aero.force_glob.R_b,aero.force_glob.Q_ref_b
  Bus Selector4 : BusSelector  OutputSignals=V_Wg_local.V_Wg_wing1,V_Wg_dt_local.V_Wg_dt_wing1
  Bus Selector5 : BusSelector  OutputSignals=envir,wind_local
  Bus Selector6 : BusSelector  OutputSignals=V_Wg_local.V_Wg_wing2,V_Wg_dt_local.V_Wg_dt_wing2
  Bus Selector7 : BusSelector  OutputSignals=V_Wg_local.V_Wg_wing3,V_Wg_dt_local.V_Wg_dt_wing3
  Bus Selector8 : BusSelector  OutputSignals=aero.R_Ab,aero.Q_Ab
  Bus Selector9 : BusSelector  OutputSignals=wing_state.aero.circulation.Gamma
  Constant1 : Constant  Value=aircraft.config.xyz_cg_c
  Constant4 : Constant  Value=0
  Constant5 : Constant  Value=abs(aircraft.wing_main.geometry.ctrl_pt.pos(2,:))<aircraft.wing_htp.params.b
  Constant6 : Constant  Value=0
  Constant8 : Constant  Value=0
  Euler Angles to Rotation Matrix : axes_transformation_lib/Euler Angles to Rotation Matrix  SystemSampleTime=-1
      settings: SourceProductName=LADAC
  Gain : Gain  Gain=aircraft.vtp_sideslip_factor
  MATLAB Function : MATLAB Function  TreatAsAtomicUnit=on
  MATLAB Function2 : MATLAB Function  TreatAsAtomicUnit=on
  MATLAB Function4 : MATLAB Function  TreatAsAtomicUnit=on
  MatrixMultiply2 : Product  Multiplication=Matrix(*)
  fuselage rigid : fuselage_lib/fuselage rigid unsteady  fuselage_struct=aircraft.fuselage  fuselage_state_bus=fuselage_1_state_bus
      settings: SourceProductName=LADAC
  unsteady downwash : wing_downwash_lib/unsteady downwash  downwash=aircraft.downwash
      settings: SourceProductName=SE2A library
  wing nlvsm : vlm_wing_lib/wing vlm rigid unsteady  wing_struct=aircraft.wing_main  wing_state_bus=wing_1_state_bus  unst_aero_state_init=0  dyn_stall_state_init=0  unst_flap_state_init=0  unst_act2_state_init=0  tau_v_init=0  alpha_ind_init=0
      settings: SourceProductName=LADAC
  wing nlvsm1 : vlm_wing_lib/wing vlm rigid unsteady  wing_struct=aircraft.wing_htp  wing_state_bus=wing_2_state_bus  unst_aero_state_init=0  dyn_stall_state_init=0  unst_flap_state_init=0  unst_act2_state_init=0  tau_v_init=0  alpha_ind_init=0
      settings: SourceProductName=LADAC
  wing nlvsm2 : vlm_wing_lib/wing vlm rigid unsteady  wing_struct=aircraft.wing_vtp  wing_state_bus=wing_3_state_bus  unst_aero_state_init=0  dyn_stall_state_init=0  unst_flap_state_init=0  unst_act2_state_init=0  tau_v_init=0  alpha_ind_init=0
      settings: SourceProductName=LADAC
  R_Ab : Outport
  Q_Ab : Outport  Port=2
  aeroBus : Outport  Port=3
  wires:
  Bus Selector8/2 -> Add1/4  "<Q_Ab>"
  Bus Selector8/1 -> Add/4  "<R_Ab>"
  Bus Selector3/2 -> Add1/3  "<Q_ref_b>"
  Bus Selector3/1 -> Add/3  "<R_b>"
  wing nlvsm2/1 -> Bus Selector3/1, Bus Creator/3  "vtp"
  pos_ref_c/1 -> wing nlvsm/9, wing nlvsm1/9, wing nlvsm2/9
  Constant8/1 -> wing nlvsm2/8
  rudder_pos/1 -> wing nlvsm2/6
  Bus Selector2/2 -> Add1/1  "<Q_ref_b>"
  Bus Selector2/1 -> Add/1  "<R_b>"
  wing nlvsm/1 -> Bus Selector2/1, Bus Selector9/1, Bus Creator/1  "main"
  Constant6/1 -> wing nlvsm/8
  actuators_pos/1 -> wing nlvsm/6
  Bus Creator/1 -> aeroBus/1  "aeroBus"
  wing nlvsm1/1 -> Bus Creator/2, Bus Selector1/1  "htp"
  htp_trim/1 -> wing nlvsm1/8
  elevator_pos/1 -> wing nlvsm1/6
  Bus Selector1/1 -> Add/2  "<R_b>"
  Bus Selector1/2 -> Add1/2  "<Q_ref_b>"
  MatrixMultiply2/1 -> Aerodynamic Angles/1
  V_Kg/1 -> MatrixMultiply2/2, MATLAB Function/1(V_A)
  Add1/1 -> Q_Ab/1
  Add/1 -> R_Ab/1
  Bus Selector5/1 -> Bus Selector/1  "<envir>"
  EulerAngles/1 -> Euler Angles to Rotation Matrix/1
  Euler Angles to Rotation Matrix/1 -> MatrixMultiply2/1
  Bus Selector7/2 -> wing nlvsm2/11  "<V_Wg_dt_wing3>"
  Bus Selector4/2 -> wing nlvsm/11  "<V_Wg_dt_wing1>"
  Bus Selector5/2 -> Bus Selector10/1, Bus Selector7/1, Bus Selector6/1, Bus Selector4/1  "<wind_local>"
  envir/1 -> Bus Selector5/1
  Bus Selector4/1 -> wing nlvsm/10  "<V_Wg_wing1>"
  Bus Selector7/1 -> wing nlvsm2/10  "<V_Wg_wing3>"
  actuators_rate/1 -> wing nlvsm/7
  elevator_rate/1 -> wing nlvsm1/7
  rudder_rate/1 -> wing nlvsm2/7
  Gain/1 -> wing nlvsm2/2
  Bus Selector10/1 -> fuselage rigid/6  "<V_Wg_fuselage>"
  omega_Kb_b/1 -> wing nlvsm1/4, fuselage rigid/4, wing nlvsm2/4, wing nlvsm/4
  Bus Selector/1 -> wing nlvsm/5, wing nlvsm1/5, fuselage rigid/8, wing nlvsm2/5  "<atmosphere>"
  Aerodynamic Angles/1 -> wing nlvsm/1, fuselage rigid/1, wing nlvsm2/1, wing nlvsm1/1
  MATLAB Function/1(V) -> wing nlvsm/3, fuselage rigid/3, wing nlvsm2/3, wing nlvsm1/3, unsteady downwash/2
  Constant1/1 -> fuselage rigid/5
  Aerodynamic Angles/2 -> wing nlvsm/2, fuselage rigid/2, Gain/1, wing nlvsm1/2
  Constant4/1 -> fuselage rigid/7
  fuselage rigid/1 -> Bus Selector8/1, Bus Creator/4  "fuselage"
  Constant5/1 -> MATLAB Function2/2(idx)
  MATLAB Function2/1(Gamma_mean) -> unsteady downwash/1  "Gamma_mean"
  Bus Selector9/1 -> MATLAB Function2/1(Gamma)  "<Gamma>"
  unsteady downwash/1 -> Bus Selector11/1, Bus Creator/5  "downwash"
  Bus Selector6/2 -> MATLAB Function4/2("V_ext_local_dt ")  "<V_Wg_dt_wing2>"
  Bus Selector6/1 -> MATLAB Function4/1("V_ext_local ")  "<V_Wg_wing2>"
  Bus Selector11/1 -> MATLAB Function4/3(w_downwash)  "<w_downwash>"
  Bus Selector11/2 -> MATLAB Function4/4(w_dt_downwash)  "<w_dt_downwash>"
  MATLAB Function4/1(V_ext_local) -> wing nlvsm1/10
  MATLAB Function4/2(V_ext_local_dt) -> wing nlvsm1/11

== matlab function flight_dynamics_models/Rigid aircraft with unsteady aerodynamics/Aerodynamics/MATLAB Function ==
  data: V_A input; V output
function V = fcn(V_A)
V = norm(V_A,2);
end

== matlab function flight_dynamics_models/Flexible aircraft with steady aerodynamics/Aerodynamics/MATLAB Function1 ==
  data: state input; pos output; vel output
function [pos,vel] = fcn(state)
len = length(state);
pos = state(1:len/2);
vel = state((len/2+1):end);
end

== matlab function flight_dynamics_models/Rigid aircraft with steady aerodynamics/Aerodynamics/MATLAB Function ==
  data: V_A input; V output
function V = fcn(V_A)
V = norm(V_A,2);
end

== matlab function flight_dynamics_models/Flexible aircraft with unsteady aerodynamics/convert aerodynamics loads and thrust to structure load/MATLAB Function2 ==
  data: R_i_Ab input; p output
function p = fcn(R_i_Ab)

p = R_i_Ab(:);

end

== matlab function flight_dynamics_models/Flexible aircraft with unsteady aerodynamics/Aerodynamics/MATLAB Function1 ==
  data: state input; pos output; vel output
function [pos,vel] = fcn(state)
len = length(state);
pos = state(1:len/2);
vel = state((len/2+1):end);
end

== matlab function flight_dynamics_models/Flexible aircraft with steady aerodynamics/Aerodynamics/MATLAB Function ==
  data: V_A input; V output
function V = fcn(V_A)
V = norm(V_A,2);
end

== matlab function flight_dynamics_models/Flexible aircraft with unsteady aerodynamics/Aerodynamics/MATLAB Function2 ==
  data: Gamma input; Gamma_mean output; idx input
function Gamma_mean = fcn(Gamma,idx)

Gamma_mean = mean( Gamma(idx) );

end

== matlab function flight_dynamics_models/Rigid aircraft with unsteady aerodynamics/Aerodynamics/MATLAB Function2 ==
  data: Gamma input; Gamma_mean output; idx input
function Gamma_mean = fcn(Gamma,idx)

Gamma_mean = mean( Gamma(idx) );

end

== matlab function flight_dynamics_models/Flexible aircraft with unsteady aerodynamics/convert aerodynamics loads and thrust to structure load/MATLAB Function3 ==
  data: R_b_i input; p output
function p = fcn(R_b_i)

p = reshape(R_b_i,[],1);

end

== matlab function flight_dynamics_models/Flexible aircraft with unsteady aerodynamics/Aerodynamics/MATLAB Function ==
  data: V_A input; V output
function V = fcn(V_A)
V = norm(V_A,2);
end

== matlab function flight_dynamics_models/Flexible aircraft with unsteady aerodynamics/Aerodynamics/MATLAB Function4 ==
  data: V_ext_local input; V_ext_local output; V_ext_local_dt input; w_downwash input; w_dt_downwash input; V_ext_local_dt output
function [V_ext_local,V_ext_local_dt] = fcn(V_ext_local,V_ext_local_dt,w_downwash, w_dt_downwash)

V_ext_local(3,:) = V_ext_local(3,:) + w_downwash;
V_ext_local_dt(3,:) = V_ext_local_dt(3,:) + w_dt_downwash;

end

== matlab function flight_dynamics_models/Rigid aircraft with unsteady aerodynamics/Aerodynamics/MATLAB Function4 ==
  data: V_ext_local input; V_ext_local output; V_ext_local_dt input; w_downwash input; w_dt_downwash input; V_ext_local_dt output
function [V_ext_local,V_ext_local_dt] = fcn(V_ext_local,V_ext_local_dt,w_downwash, w_dt_downwash)

V_ext_local(3,:) = V_ext_local(3,:) + w_downwash;
V_ext_local_dt(3,:) = V_ext_local_dt(3,:) + w_dt_downwash;

end

== matlab function flight_dynamics_models/Flexible aircraft with unsteady aerodynamics/Propulsion/MATLAB Function1 ==
  data: R_b_i output; thrust input; eta input; pos_ref_c input; R_b output; Q_b output; engines parameter
function [R_b_i,R_b,Q_b] = enginesGetLoads(thrust,eta,pos_ref_c, engines)
[R_b_i,R_b,Q_b] = enginesGetLoads(engines,thrust,eta,pos_ref_c);
end

== matlab function flight_dynamics_models/Flexible aircraft with unsteady aerodynamics/convert aerodynamics loads and thrust to structure load/MATLAB Function1 ==
  data: R_i_Ab input; M_profile_i_Ab input; p output
function p = fcn(R_i_Ab, M_profile_i_Ab)

p = reshape([R_i_Ab;M_profile_i_Ab],[],1);

end

== matlab function flight_dynamics_models/Flexible aircraft with unsteady aerodynamics/convert aerodynamics loads and thrust to structure load/MATLAB Function7 ==
  data: R_i_Ab input; M_profile_i_Ab input; p output
function p = fcn(R_i_Ab, M_profile_i_Ab)

p = reshape([R_i_Ab;M_profile_i_Ab],[],1);

end

== matlab function flight_dynamics_models/Flexible aircraft with unsteady aerodynamics/convert aerodynamics loads and thrust to structure load/MATLAB Function8 ==
  data: R_i_Ab input; M_profile_i_Ab input; p output
function p = fcn(R_i_Ab, M_profile_i_Ab)

p = reshape([R_i_Ab;M_profile_i_Ab],[],1);

end

== matlab function flight_dynamics_models/Flexible aircraft with steady aerodynamics/Aerodynamics/MATLAB Function2 ==
  data: Gamma input; Gamma_mean output; idx input
function Gamma_mean = fcn(Gamma,idx)

Gamma_mean = mean( Gamma(idx) );

end

== matlab function flight_dynamics_models/Flexible aircraft with steady aerodynamics/Aerodynamics/MATLAB Function4 ==
  data: V_ext_local input; V_ext_local output; w_downwash input
function V_ext_local  = fcn(V_ext_local ,w_downwash)

V_ext_local(3,:) = V_ext_local(3,:) + w_downwash;

end

== matlab function flight_dynamics_models/Rigid aircraft with steady aerodynamics/Aerodynamics/MATLAB Function2 ==
  data: Gamma input; Gamma_mean output; idx input
function Gamma_mean = fcn(Gamma,idx)

Gamma_mean = mean( Gamma(idx) );

end
